simulink model "Simulation"  (R2021b)
settings: Solver=VariableStepAuto  StartTime=0.0  StopTime=10.0  RelTol=1e-3
undefined symbols (not defined in the file): Ad, Bd, Cd, K, kr, L, Ts
libraries: cstblocks x1
settings Model: Creator=UTENTE  LastModifiedBy=UTENTE

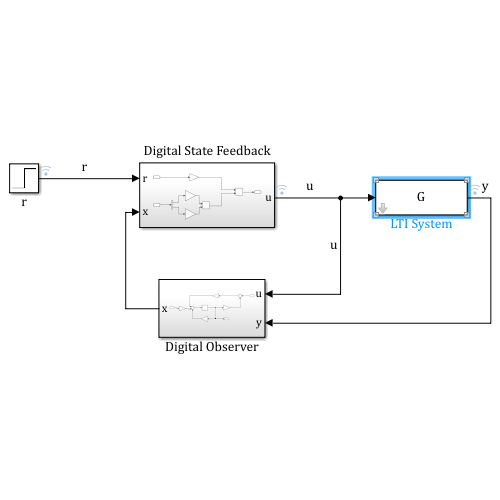
[thumbnail: Simulink's stored preview of the top-level diagram]
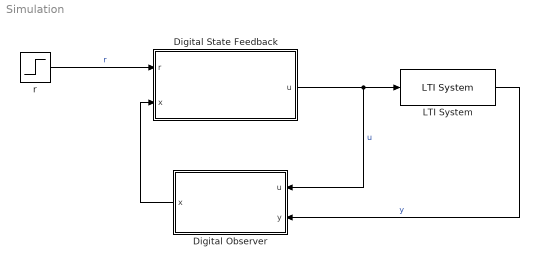
== system Simulation ==
  Digital Observer : Subsystem
  Digital State Feedback : Subsystem
  LTI System : cstblocks/LTI System  sys=G  IC=[]
  r : Step  After=10  SampleTime=Ts
  wires:
  LTI System/1 -> Digital Observer/2(y)  "y"
  Digital State Feedback/1(u) -> Digital Observer/1(u), LTI System/1  "u"
  r/1 -> Digital State Feedback/1(r)  "r"
  Digital Observer/1(x) -> Digital State Feedback/2(x)

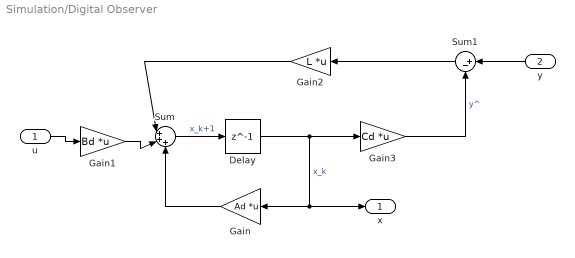
== system Simulation/Digital Observer ==
  u : Inport
  y : Inport  Port=2
  Delay : Delay  DelayLength=1  SampleTime=Ts
  Gain : Gain  Gain=Ad  Multiplication=Matrix(K*u)
  Gain1 : Gain  Gain=Bd  Multiplication=Matrix(K*u)
  Gain2 : Gain  Gain=L  Multiplication=Matrix(K*u)
  Gain3 : Gain  Gain=Cd  Multiplication=Matrix(K*u)
  Sum : Sum  Inputs=|+++
  Sum1 : Sum  Inputs=|+-
  x : Outport
  wires:
  u/1 -> Gain1/1
  Gain3/1 -> Sum1/2  "y^"
  Delay/1 -> x/1, Gain/1, Gain3/1  "x_k"
  Gain1/1 -> Sum/2
  Gain2/1 -> Sum/1
  Sum/1 -> Delay/1  "x_k+1"
  Gain/1 -> Sum/3
  Sum1/1 -> Gain2/1
  y/1 -> Sum1/1

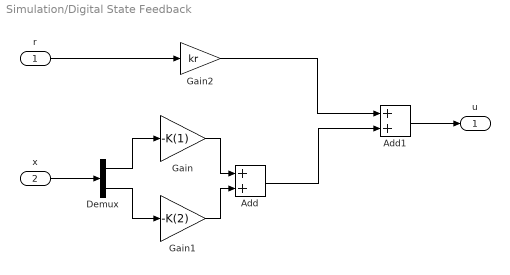
== system Simulation/Digital State Feedback ==
  r : Inport
  x : Inport  Port=2
  Add : Sum
  Add1 : Sum
  Demux : Demux  Outputs=2
  Gain : Gain  Gain=-K(1)
  Gain1 : Gain  Gain=-K(2)
  Gain2 : Gain  Gain=kr
  u : Outport
  wires:
  Demux/2 -> Gain1/1
  Gain1/1 -> Add/2
  Add/1 -> Add1/2
  Add1/1 -> u/1
  Gain/1 -> Add/1
  Demux/1 -> Gain/1
  x/1 -> Demux/1
  r/1 -> Gain2/1
  Gain2/1 -> Add1/1
